simulink model "PlatGoughStewart"  (R2017b)
settings: Solver=ode45  StartTime=0.0  StopTime=5  MaxStep=0.2  RelTol=1e-3
settings Model: Creator=Enrique Benavides  LastModifiedBy=Enrique Benavides

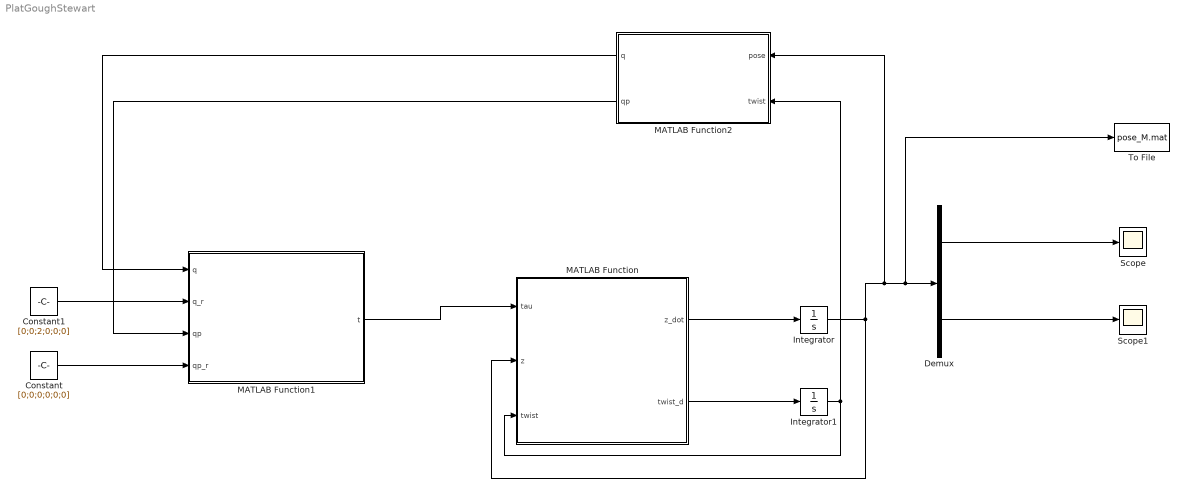
== system PlatGoughStewart ==
  Constant : Constant  Value=[0;0;0;0;0;0]
  Constant1 : Constant  Value=[0;0;2;0;0;0]
  Demux : Demux  Outputs=2
  Integrator : Integrator  InitialCondition=[0;0;3;0;0;0]
  Integrator1 : Integrator  InitialCondition=[0;0;0;0;0;0]
  MATLAB Function : MATLAB Function  TreatAsAtomicUnit=on
  MATLAB Function1 : MATLAB Function  TreatAsAtomicUnit=on
  MATLAB Function2 : MATLAB Function  TreatAsAtomicUnit=on
  Scope : Scope
  Scope1 : Scope
  To File : ToFile  Filename=pose_M.mat  MatrixName=pose  SaveFormat=Timeseries
  wires:
  MATLAB Function/1(z_dot) -> Integrator/1
  MATLAB Function/2(twist_d) -> Integrator1/1
  Integrator1/1 -> MATLAB Function/3(twist), MATLAB Function2/2(twist)
  Integrator/1 -> MATLAB Function2/1(pose), To File/1, Demux/1, MATLAB Function/2(z)
  Demux/1 -> Scope/1
  Demux/2 -> Scope1/1
  MATLAB Function1/1(t) -> MATLAB Function/1(tau)
  MATLAB Function2/1(q) -> MATLAB Function1/1(q)
  MATLAB Function2/2(qp) -> MATLAB Function1/3(qp)
  Constant/1 -> MATLAB Function1/4(qp_r)
  Constant1/1 -> MATLAB Function1/2(q_r)

== matlab function PlatGoughStewart/MATLAB Function1 ==
  data: q input; q_r input; t output; qp input; qp_r input
function t = fcn(q,q_r,qp,qp_r)

eq = q - q_r;
eqp = qp - qp_r;

k_p = [10,10,10,10,10,10];
k_v = [.1,.1,.1,.1,.1,.1];
t = zeros(6,1);

for i = 1:6
  t(i,1) = k_p(i)*eq(i) + eqp(i)*k_v(i);
end

end

== matlab function PlatGoughStewart/MATLAB Function ==
  data: tau input; z_dot output; twist_d output; z input; twist input
function [z_dot,twist_d] = fcn(tau,z,twist)
[anga,angb,a,b,lmin] = plat_prop();

% Prealocacion de las variables
d = zeros(3,1); R_ang = zeros(3,1);

% Variables de entrada
d(:,1) = z(1:3);
R_ang(:,1) = z(4:6);
b_f = [.1;.1;.1;.1;.1;.1];

% Matriz de rotacion de la plataforma
MRot = M_Rot(R_ang(3),'z','r')*M_Rot(R_ang(2),'y','r')*M_Rot(R_ang(1),'x','r');

[lam,th_i] = p_IK(d,R_ang,anga,angb,a,b);

% Obtener pseudo-Cinematica velocidad
[X_p,Jac,t_dot] = p_IVK(th_i,anga,angb,a,b,MRot,lam,lmin,twist);

% Obtener quasi lagarangiano
twist_d = Q_LIK(Jac,t_dot,X_p,twist,lam,tau,b_f,MRot,a);
z_dot = inv(op_cin(R_ang))*twist;

end

== matlab function PlatGoughStewart/MATLAB Function2 ==
  data: pose input; q output; twist input; qp output
function [q,qp] = fcn(pose,twist)
d = pose(1:3);
R = Rotz(pose(6))*Roty(pose(5))*Rotx(pose(4));

[anga,angb,a,b,lmin] = plat_prop();
l = zeros(3,6);
q = zeros(6,1);
lam = zeros(3,6);

for i = 1:6
    l(:,i) = d + R*a(:,i) - b(:,i);
    q(i)=norm(l(:,i));
    lam(:,i) = l(:,i)/q(i);
end

A = zeros(6,6);
for i = 1:6
    A(i,1:3) = lam(:,i)';
    d = R*a(:,i);
    cc = cross(d,lam(:,i));
    A(i,4:6) = cc';
end

qp = A*twist;

end
